simulink model "ZVDshaper"  (R2018b)
settings: Solver=VariableStepAuto  StartTime=0.0  StopTime=.05  MaxStep=1E-6  RelTol=1E-5
libraries: simulink x1
settings Model: Creator=Biao Cheng  LastModifiedBy=ohara

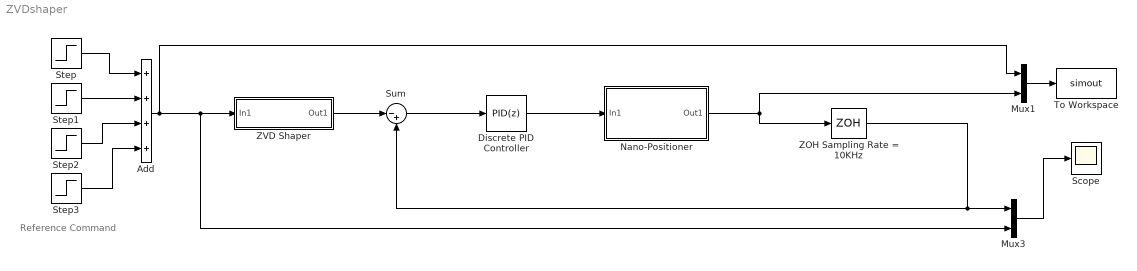
== system ZVDshaper ==
  note: Reference Command
  Add : Sum  Inputs=++++
  Discrete PID Controller : simulink/Continuous/PID Controller  Controller=PID  Form=Parallel  TimeDomain=Discrete-time  SampleTime=-1  IntegratorMethod=Forward Euler  FilterMethod=Forward Euler  ControllerParametersSource=internal  P=-0.458017813135217  I=-1774.5406525772  D=-2.81107720895671e-05  UseFilter=on  N=162369.527803254  TunerSelectOption=Transfer Function Based (PID Tuner App)  InitialConditionSource=internal  InitialConditionForIntegrator=0  InitialConditionForFilter=0  DifferentiatorICPrevScaledInput=0  ExternalReset=none  TrackingMode=off  Kt=1  LimitOutput=off  UpperSaturationLimit=inf  LowerSaturationLimit=-inf  LinearizeAsGain=off  AntiWindupMode=none  Kb=1  POutMin=[]  POutMax=[]  IOutMin=[]  IOutMax=[]  DOutMin=[]  DOutMax=[]  NOutMin=[]  NOutMax=[]  SumOutMin=[]  SumOutMax=[]  SaturationOutMin=[]  SaturationOutMax=[]  PParamMin=[]  PParamMax=[]  IParamMin=[]  IParamMax=[]  DParamMin=[]  DParamMax=[]  NParamMin=[]  NParamMax=[]  KbParamMin=[]  KbParamMax=[]  KtParamMin=[]  KtParamMax=[]  KbOutMin=[]  KbOutMax=[]  KtOutMin=[]  KtOutMax=[]  IntegratorOutMin=[]  IntegratorOutMax=[]  FilterOutMin=[]  FilterOutMax=[]  SumI1OutMin=[]  SumI1OutMax=[]  SumI2OutMin=[]  SumI2OutMax=[]  SumI3OutMin=[]  SumI3OutMax=[]  SumI4OutMin=[]  SumI4OutMax=[]  SumDOutMin=[]  SumDOutMax=[]  DifferentiatorOutMin=[]  DifferentiatorOutMax=[]  FilterDiffOutCoefMin=[]  FilterDiffOutCoefMax=[]  ReciprocalOutMin=[]  ReciprocalOutMax=[]  SumDenOutMin=[]  SumDenOutMax=[]  SumNumOutMin=[]  SumNumOutMax=[]  DivideOutMin=[]  DivideOutMax=[]  IntegratorContinuousStateAttributes=''  IntegratorStateMustResolveToSignalObject=off  IntegratorRTWStateStorageClass=Auto  FilterContinuousStateAttributes=''  FilterStateMustResolveToSignalObject=off  FilterRTWStateStorageClass=Auto  ParallelPVariant=InternalParameters  IdealPVariant=Disabled  IVariant=InternalParameters  DVariant=InternalParameters  IntegratorVariant=Discrete  SatVariant=Disabled  AWVariant=Passthrough  PCopyVariant=Disabled  TRVariant=Disabled  FdbkBlocksVariant=Forward  IdealPFdbkVariant=Disabled  SatFdbkVariant=Disabled  DerivativeFilterVariant=ForwardEulerFilter  NVariant=InternalParameters  NCopyVariant=Disabled  FilterICVariant=InternalICsFilter  IntegratorICVariant=InternalICs  ExternalResetVariant=Disabled  TRSumVariant=Passthrough  SumFdbkVariant=Disabled  SumVariant=Sum_PID
  Mux1 : Mux  Inputs=2
  Mux3 : Mux  Inputs=2
  Nano-Positioner : Subsystem
  Scope : Scope
  Step : Step  Time=5E-3  SampleTime=0
  Step1 : Step  Time=15E-3  SampleTime=0
  Step2 : Step  Time=25E-3  After=-1  SampleTime=0
  Step3 : Step  Time=35E-3  After=-1  SampleTime=0
  Sum : Sum  Inputs=|-+
  To Workspace : ToWorkspace  VariableName=simout  SaveFormat=Timeseries  SampleTime=1/10000
  ZOH Sampling Rate = 10KHz : ZeroOrderHold  SampleTime=1E-5
  "ZVD Shaper " : Subsystem
  wires:
  Step/1 -> Add/1
  Step1/1 -> Add/2
  Step2/1 -> Add/3
  Step3/1 -> Add/4
  Nano-Positioner/1(Out1) -> ZOH Sampling Rate = 10KHz/1, Mux1/2
  Mux1/1 -> To Workspace/1
  Sum/1 -> Discrete PID Controller/1
  ZOH Sampling Rate = 10KHz/1 -> Sum/2, Mux3/1
  Mux3/1 -> Scope/1
  Add/1 -> "ZVD Shaper "/1(In1), Mux3/2, Mux1/1
  Discrete PID Controller/1 -> Nano-Positioner/1(In1)
  "ZVD Shaper "/1(Out1) -> Sum/1

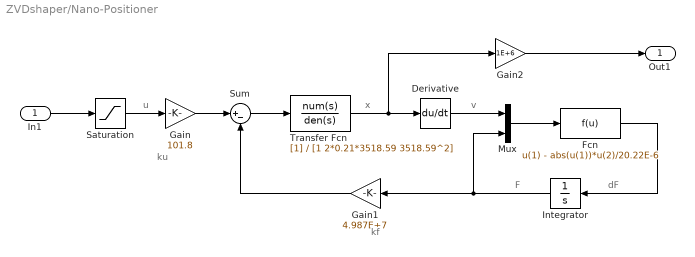
== system ZVDshaper/Nano-Positioner ==
  note: dF
  note: F
  note: v
  note: x
  note: kf
  note: u
  note: ku
  In1 : Inport
  Derivative : Derivative
  Fcn : Fcn  Expr=u(1) - abs(u(1))*u(2)/20.22E-6
  Gain : Gain  Gain=101.8
  Gain1 : Gain  Gain=4.987E+7
  Gain2 : Gain  Gain=1E+6
  Integrator : Integrator
  Mux : Mux  Inputs=2
  Saturation : Saturate  UpperLimit=4  LowerLimit=-4
  Sum : Sum  Inputs=|+-
  Transfer Fcn : TransferFcn  Denominator=[1 2*0.21*3518.59 3518.59^2]
  Out1 : Outport
  wires:
  Gain1/1 -> Sum/2
  Mux/1 -> Fcn/1
  Integrator/1 -> Mux/2, Gain1/1
  In1/1 -> Saturation/1
  Derivative/1 -> Mux/1
  Fcn/1 -> Integrator/1
  Sum/1 -> Transfer Fcn/1
  Saturation/1 -> Gain/1
  Gain/1 -> Sum/1
  Transfer Fcn/1 -> Gain2/1, Derivative/1
  Gain2/1 -> Out1/1

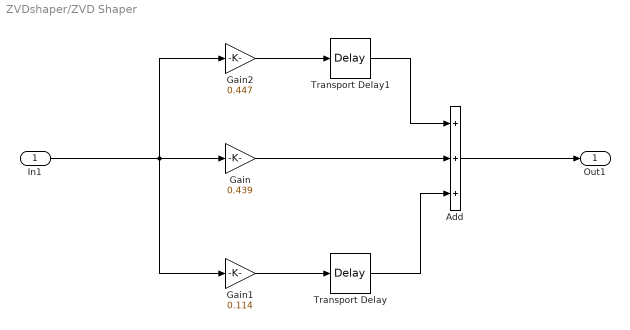
== system ZVDshaper/ZVD Shaper  ==
  In1 : Inport
  Add : Sum  Inputs=+++
  Gain : Gain  Gain=0.439
  Gain1 : Gain  Gain=0.114
  Gain2 : Gain  Gain=0.447
  Transport Delay : TransportDelay  DelayTime=1E-3
  Transport Delay1 : TransportDelay  DelayTime=1E-3
  Out1 : Outport
  wires:
  Gain1/1 -> Transport Delay/1
  Transport Delay/1 -> Add/3
  Gain/1 -> Add/2
  Add/1 -> Out1/1
  In1/1 -> Gain1/1, Gain/1, Gain2/1
  Gain2/1 -> Transport Delay1/1
  Transport Delay1/1 -> Add/1
